simulink model "MPTC_TR"  (R2019b)
settings: Solver=ode4  StartTime=0.0  StopTime=1  FixedStep=1e-6  RelTol=1e-3  EnableMultiTasking=on
values from neighbouring files (symbols this model uses):
  B = 0    [Parameters_MPC.m]
  J = 0.0165    [Parameters_MPC.m]
  kr = (Lm/Lr)    (= 0.960714285714)    [Parameters_MPC.m]
  Lm = 0.0538    [Parameters_MPC.m]
  P = 2    [Parameters_MPC.m]
  r_sigma = Rs+Rr*(kr^2)    (= 0.445903864796)    [Parameters_MPC.m]
  Rs = 0.277    [Parameters_MPC.m]
  set_speed = 500    [Parameters_MPC.m]
  t_sigma = (sigma*Ls)/(r_sigma)    (= 0.00810392489023)    [Parameters_MPC.m]
  tr = Lr/Rr    (= 0.306010928962)    [Parameters_MPC.m]
libraries: powerlib_meascontrol x6, simulink x2, powerlib x1
settings Model: Creator=91913  LastModifiedBy=akhil
settings SolverCC: PositivePriorityOrder=on  AutoInsertRateTranBlk=on
settings DataIOCC: SaveOutput=off  DSMLogging=off  ReturnWorkspaceOutputs=off  SignalLoggingName=logsout_MPTCTR

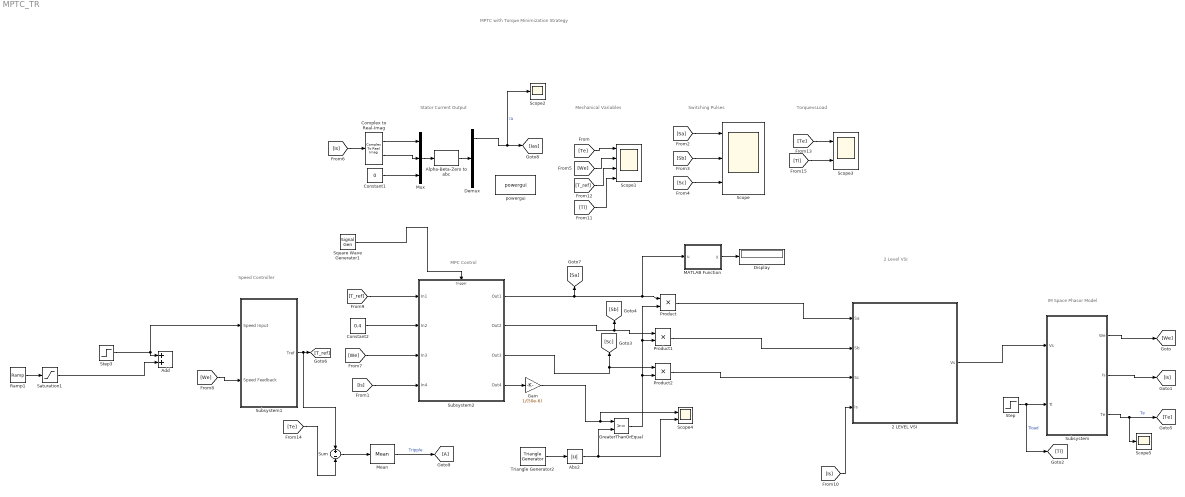
== system MPTC_TR ==
  note: MPTC with Torque Minimization Strategy
  note: IM Space Phasor Model
  note: 2 Level VSI
  note: Mechanical Variables
  note: Switching Pulses
  note: Speed Controller
  note: MPC Control
  note: Stator Current Output
  note: TorquevsLoad
  2 LEVEL VSI : Subsystem
  Abs2 : Abs
  Add : Sum
  Alpha-Beta-Zero to abc : powerlib_meascontrol/Transformations/Alpha-Beta-Zero to abc
      settings: SourceProductName=Simscape Electrical  SourceProductBaseCode=PS
  Complex to Real-Imag : ComplexToRealImag
  Constant1 : Constant  Value=0
  Constant2 : Constant  Value=0.4
  Demux : Demux  Outputs=3
  Display : Display
  Gain : Gain  Gain=1/(50e-6)
  GreaterThanOrEqual : RelationalOperator  OutDataTypeStr=boolean  RndMeth=Simplest
  MATLAB Function : MATLAB Function  TreatAsAtomicUnit=on
  Mean : powerlib_meascontrol/Measurements/Mean  Freq=41  Vinit=0  Ts=0
      settings: SourceProductName=Simscape Electrical
  Mux : Mux  Inputs=3
  Product : Product
  Product1 : Product
  Product2 : Product
  Ramp1 : simulink/Sources/Ramp  slope=-2*set_speed  start=0.4  InitialOutput=0
  Saturation1 : Saturate  UpperLimit=0  LowerLimit=-200
  Scope : Scope  NumInputPorts=3
  Scope1 : Scope  NumInputPorts=4
  Scope2 : Scope
  Scope3 : Scope  NumInputPorts=2
  Scope4 : Scope  NumInputPorts=2
  Scope5 : Scope
  Square Wave Generator1 : SignalGenerator  WaveForm=square  Frequency=1/(50e-6)
  Step : Step  Time=0.5  After=20  SampleTime=0
  Step3 : Step  Time=0.1  After=set_speed  SampleTime=0
  Subsystem : Subsystem
  Subsystem1 : Subsystem
  Subsystem2 : Subsystem
  Sum : Sum  Inputs=+-
  Triangle Generator2 : powerlib_meascontrol/Pulse & Signal Generators/Triangle Generator  Freq=5e4  Phase=90  Ts=0
      settings: SourceProductName=Simscape Electrical
  powergui : powerlib/powergui  Priority=1  SimulationMode=Continuous  SampleTime=50e-6  frequency=60  Iterations=50  frequencyindice=60  Pbase=100e6  ErrMax=1e-4  UnitsV=kV  UnitsW=MW  buscounter=0  FunctionMessages=off  echomessages=off  EnableUseOfTLC=off  CurrentSourceSwitches=off  DisableSnubberDevices=off  DisableRonSwitches=off  DisableVfSwitches=off  DisplayEquations=off  AutomaticDiscreteSolvers=off  SolverType=Tustin/Backward Euler (TBE)  Interpol=off  ExternalGateDelay=off  methode=off  Ts=100  x0status=blocks  SPID=on  SwTol=0  HookPort=off  NonlinearTolerance=1e-4  nMaxIteration=100  ContinueOnMaxIteration=off  RestoreLinks=warning  ResistiveCurrentMeasurement=off  Frange=[0:2:500]  Ylog=off  Xlog=on  ShowGrid=off  save=off  variable=ZData  structure=logsout  ZoomFFT=off  StartTime=1.2  cycles=20  DisplayStyle=1  fundamental=49.3  FreqAxis=on  MaxFrequency=1000  frequencyindicesteady=1  RmsSteady=1  display=off
      settings: SourceProductName=Simscape Electrical
  wires:
  2 LEVEL VSI/1(Vs) -> Subsystem/1(Vs)
  Gain/1 -> Scope4/1, GreaterThanOrEqual/1
  Square Wave Generator1/1 -> Subsystem2/Trigger
  [Tl] -> Scope3/2
  Subsystem/3(Te) -> Scope5/1, [Te]  "Te"
  Step/1 -> [Tl], Subsystem/2(Tl)  "Tload"
  Product/1 -> 2 LEVEL VSI/1(Sa)
  Triangle Generator2/1 -> Abs2/1
  Product1/1 -> 2 LEVEL VSI/2(Sb)
  Subsystem/1(We) -> [We]
  Subsystem2/4(Out4) -> Gain/1
  [Te] -> Scope3/1
  [Sc] -> Scope/3
  Subsystem2/2(Out2) -> Product1/1, [Sb]
  Product2/1 -> 2 LEVEL VSI/3(Sc)
  GreaterThanOrEqual/1 -> Product/2, Product1/2, Product2/2
  Constant1/1 -> Mux/3
  [Te] -> Scope1/1
  Subsystem2/3(Out3) -> [Sc], Product2/1
  Subsystem2/1(Out1) -> MATLAB Function/1(u), Product/1, [Sa]
  [Is] -> Subsystem2/4(In4)
  Complex to Real-Imag/2 -> Mux/2
  [Is] -> Complex to Real-Imag/1
  [Sa] -> Scope/1
  [We] -> Subsystem2/3(In3)
  Complex to Real-Imag/1 -> Mux/1
  Subsystem/2(Is) -> [Is]
  Abs2/1 -> Scope4/2, GreaterThanOrEqual/2
  [We] -> Scope1/2
  Alpha-Beta-Zero to abc/1 -> Demux/1
  [Tl] -> Scope1/4
  Subsystem1/1(Tref) -> Sum/1, [T_ref]
  Mux/1 -> Alpha-Beta-Zero to abc/1
  [We] -> Subsystem1/2(Speed Feedback)
  [T_ref] -> Scope1/3
  [Sb] -> Scope/2
  [Is] -> 2 LEVEL VSI/4(Is)
  Constant2/1 -> Subsystem2/2(In2)
  Demux/1 -> Scope2/1, [Ias]  "Ia"
  [Te] -> Sum/2
  Sum/1 -> Mean/1
  Mean/1 -> [A]  "Tripple"
  [T_ref] -> Subsystem2/1(In1)
  MATLAB Function/1(y) -> Display/1
  Step3/1 -> Subsystem1/1(Speed Input), Add/1
  Saturation1/1 -> Add/2
  Ramp1/1 -> Saturation1/1

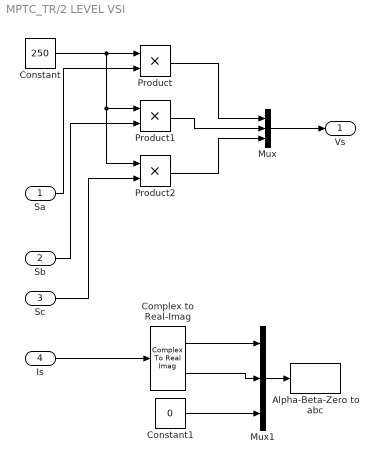
== system MPTC_TR/2 LEVEL VSI ==
  Sa : Inport
  Sb : Inport  Port=2
  Sc : Inport  Port=3
  Is : Inport  Port=4
  Alpha-Beta-Zero to abc : powerlib_meascontrol/Transformations/Alpha-Beta-Zero to abc
      settings: SourceProductName=Simscape Electrical  SourceProductBaseCode=PS
  Complex to Real-Imag : ComplexToRealImag
  Constant : Constant  Value=250
  Constant1 : Constant  Value=0
  Mux : Mux  Inputs=3
  Mux1 : Mux  Inputs=3
  Product : Product
  Product1 : Product
  Product2 : Product
  Vs : Outport
  wires:
  Sa/1 -> Product/2
  Sb/1 -> Product1/2
  Sc/1 -> Product2/2
  Constant/1 -> Product2/1, Product1/1, Product/1
  Product/1 -> Mux/1
  Product1/1 -> Mux/2
  Product2/1 -> Mux/3
  Mux/1 -> Vs/1
  Complex to Real-Imag/1 -> Mux1/1
  Complex to Real-Imag/2 -> Mux1/2
  Constant1/1 -> Mux1/3
  Mux1/1 -> Alpha-Beta-Zero to abc/1
  Is/1 -> Complex to Real-Imag/1

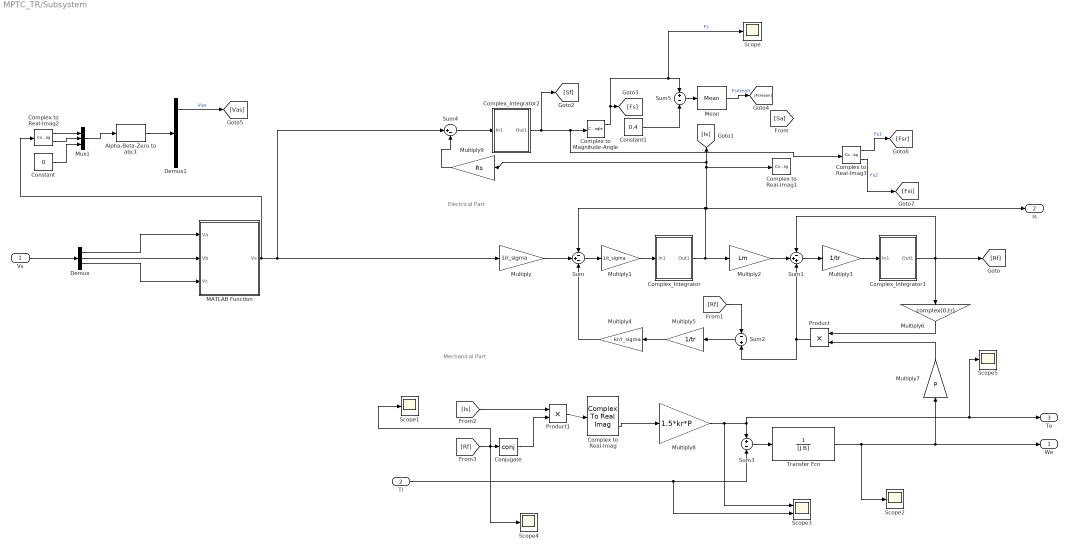
== system MPTC_TR/Subsystem ==
  note: Mechanical Part
  note: Electrical Part
  Vs : Inport
  Tl : Inport  Port=2
  Alpha-Beta-Zero to abc1 : powerlib_meascontrol/Transformations/Alpha-Beta-Zero to abc
      settings: SourceProductName=Simscape Electrical  SourceProductBaseCode=PS
  Complex to Magnitude-Angle : ComplexToMagnitudeAngle
  Complex to Real-Imag{,1..3} (4 alike) : ComplexToRealImag
  Complex_Integrator : Subsystem
  Complex_Integrator1 : Subsystem
  Complex_Integrator2 : Subsystem
  Conjugate : Math  Operator=conj  RndMeth=Zero  SaturateOnIntegerOverflow=on
  Constant : Constant  Value=0
  Constant1 : Constant  Value=0.4
  Demux : Demux  Outputs=3
  Demux1 : Demux  Outputs=3
  MATLAB Function : MATLAB Function  TreatAsAtomicUnit=on
  Mean : powerlib_meascontrol/Measurements/Mean  Freq=41  Vinit=0  Ts=0
      settings: SourceProductName=Simscape Electrical
  Multiply : Gain  Gain=1/r_sigma
  Multiply1 : Gain  Gain=1/t_sigma
  Multiply2 : Gain  Gain=Lm
  Multiply3 : Gain  Gain=1/tr
  Multiply4 : Gain  Gain=kr/r_sigma
  Multiply5 : Gain  Gain=1/tr
  Multiply6 : Gain  Gain=complex(0,tr)
  Multiply7 : Gain  Gain=P
  Multiply8 : Gain  Gain=1.5*kr*P
  Multiply9 : Gain  Gain=Rs
  Mux1 : Mux  Inputs=3
  Product : Product
  Product1 : Product
  Scope{,1..2,4..5} (5 alike) : Scope
  Scope3 : Scope  NumInputPorts=2
  Sum : Sum  Inputs=-+-
  Sum1 : Sum  Inputs=-++
  Sum2 : Sum  Inputs=-+
  Sum3 : Sum  Inputs=+-
  Sum4 : Sum  Inputs=|+-
  Sum5 : Sum  Inputs=+-
  Transfer Fcn : TransferFcn  Denominator=[J B]
  We : Outport
  Is : Outport  Port=2
  Te : Outport  Port=3
  wires:
  [Is] -> Product1/1
  Multiply1/1 -> Complex_Integrator/1(In1)
  Multiply4/1 -> Sum/3
  Multiply3/1 -> Complex_Integrator1/1(In1)
  Sum1/1 -> Multiply3/1
  Complex to Real-Imag/2 -> Multiply8/1
  Complex_Integrator1/1(Out1) -> Sum1/1, [Rf], Multiply6/1
  Tl/1 -> Scope3/2, Sum3/2
  Conjugate/1 -> Product1/2
  Multiply7/1 -> Product/2
  Multiply8/1 -> Scope3/1, Sum3/1, Scope5/1, Te/1
  Multiply2/1 -> Sum1/2
  Multiply/1 -> Sum/2
  Multiply6/1 -> Product/1
  Product/1 -> Sum2/2, Sum1/3
  Multiply5/1 -> Multiply4/1
  Sum2/1 -> Multiply5/1
  Transfer Fcn/1 -> Scope2/1, We/1, Multiply7/1
  Sum/1 -> Multiply1/1
  [Rf] -> Scope1/1, Conjugate/1, Scope4/1
  Product1/1 -> Complex to Real-Imag/1
  Sum3/1 -> Transfer Fcn/1
  [Rf] -> Sum2/1
  Sum4/1 -> Complex_Integrator2/1(In1)
  Complex_Integrator2/1(Out1) -> Complex to Real-Imag3/1, Complex to Magnitude-Angle/1, [Sf]
  Multiply9/1 -> Sum4/2
  Complex_Integrator/1(Out1) -> Multiply2/1, Multiply9/1, [Is], Complex to Real-Imag1/1, Is/1, Sum/1
  MATLAB Function/1(Vs) -> Complex to Real-Imag2/1, Sum4/1, Multiply/1
  Vs/1 -> Demux/1
  Demux/1 -> MATLAB Function/1(Va)
  Demux/2 -> MATLAB Function/2(Vb)
  Demux/3 -> MATLAB Function/3(Vc)
  Constant/1 -> Mux1/3
  Alpha-Beta-Zero to abc1/1 -> Demux1/1
  Mux1/1 -> Alpha-Beta-Zero to abc1/1
  Complex to Real-Imag2/2 -> Mux1/2
  Complex to Real-Imag2/1 -> Mux1/1
  Complex to Magnitude-Angle/1 -> Scope/1, Sum5/1, [Fs]  "Fs"
  Constant1/1 -> Sum5/2
  Sum5/1 -> Mean/1
  Mean/1 -> [Fsmean]  "Fsmean"
  Demux1/1 -> [Vas]  "Vas"
  Complex to Real-Imag3/2 -> [Fsi]  "Fs2"
  Complex to Real-Imag3/1 -> [Fsr]  "Fs1"

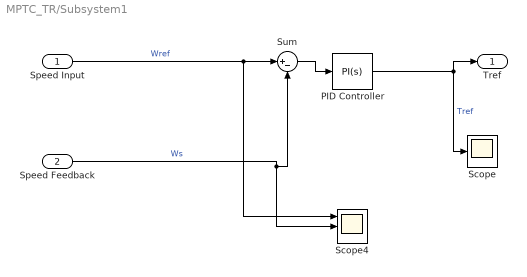
== system MPTC_TR/Subsystem1 ==
  Speed Input : Inport
  Speed Feedback : Inport  Port=2
  PID Controller : simulink/Continuous/PID Controller  Controller=PI  Form=Parallel  TimeDomain=Continuous-time  SampleTime=-1  IntegratorMethod=Forward Euler  FilterMethod=Forward Euler  ControllerParametersSource=internal  P=100  I=2000  D=0  UseFilter=on  N=100  TunerSelectOption=Transfer Function Based (PID Tuner App)  InitialConditionSource=internal  InitialConditionForIntegrator=0  InitialConditionForFilter=0  DifferentiatorICPrevScaledInput=0  ExternalReset=none  TrackingMode=off  Kt=1  LimitOutput=on  UpperSaturationLimit=75  LowerSaturationLimit=-75  LinearizeAsGain=off  AntiWindupMode=clamping  Kb=1  POutMin=[]  POutMax=[]  IOutMin=[]  IOutMax=[]  DOutMin=[]  DOutMax=[]  NOutMin=[]  NOutMax=[]  SumOutMin=[]  SumOutMax=[]  SaturationOutMin=[]  SaturationOutMax=[]  PParamMin=[]  PParamMax=[]  IParamMin=[]  IParamMax=[]  DParamMin=[]  DParamMax=[]  NParamMin=[]  NParamMax=[]  KbParamMin=[]  KbParamMax=[]  KtParamMin=[]  KtParamMax=[]  KbOutMin=[]  KbOutMax=[]  KtOutMin=[]  KtOutMax=[]  IntegratorOutMin=[]  IntegratorOutMax=[]  FilterOutMin=[]  FilterOutMax=[]  SumI1OutMin=[]  SumI1OutMax=[]  SumI2OutMin=[]  SumI2OutMax=[]  SumI3OutMin=[]  SumI3OutMax=[]  SumI4OutMin=[]  SumI4OutMax=[]  SumDOutMin=[]  SumDOutMax=[]  DifferentiatorOutMin=[]  DifferentiatorOutMax=[]  FilterDiffOutCoefMin=[]  FilterDiffOutCoefMax=[]  ReciprocalOutMin=[]  ReciprocalOutMax=[]  SumDenOutMin=[]  SumDenOutMax=[]  SumNumOutMin=[]  SumNumOutMax=[]  DivideOutMin=[]  DivideOutMax=[]  IntegratorContinuousStateAttributes=''  IntegratorStateMustResolveToSignalObject=off  IntegratorRTWStateStorageClass=Auto  FilterContinuousStateAttributes=''  FilterStateMustResolveToSignalObject=off  FilterRTWStateStorageClass=Auto  ParallelPVariant=InternalParameters  IdealPVariant=Disabled  IVariant=InternalParameters  DVariant=Disabled  IntegratorVariant=Continuous  SatVariant=Enabled  AWVariant=ContClampingParallel  PCopyVariant=Disabled  TRVariant=Disabled  FdbkBlocksVariant=Forward  IdealPFdbkVariant=Disabled  SatFdbkVariant=Disabled  DerivativeFilterVariant=Disabled  NVariant=Disabled  NCopyVariant=Disabled_SignalSpec  FilterICVariant=Disabled  IntegratorICVariant=InternalICs  ExternalResetVariant=Disabled  TRSumVariant=Passthrough  SumFdbkVariant=Disabled  SumVariant=Sum_PI
  Scope : Scope
  Scope4 : Scope  NumInputPorts=3
  Sum : Sum  Inputs=|+-
  Tref : Outport
  wires:
  Speed Input/1 -> Scope4/1, Sum/1  "Wref"
  Speed Feedback/1 -> Scope4/2, Sum/2  "Ws"
  Sum/1 -> PID Controller/1
  PID Controller/1 -> Tref/1, Scope/1  "Tref"

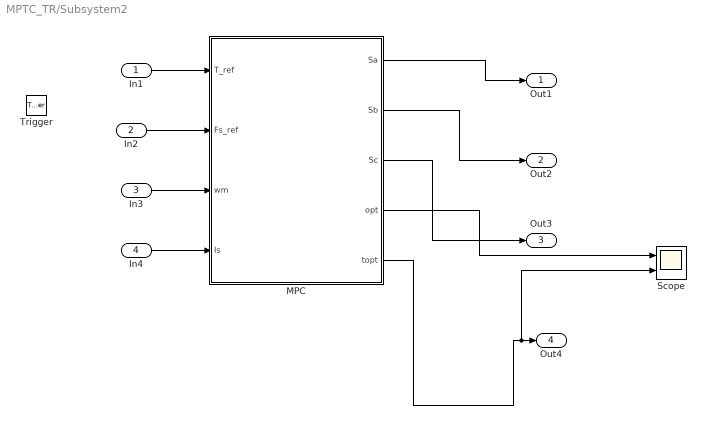
== system MPTC_TR/Subsystem2 ==
  In1 : Inport
  In2 : Inport  Port=2
  In3 : Inport  Port=3
  In4 : Inport  Port=4
  Trigger : TriggerPort  VariantControl=Variant  ShowOutputPort=on  PortDimensions=1
  MPC : MATLAB Function  TreatAsAtomicUnit=on
  Scope : Scope  NumInputPorts=2
  Out1 : Outport
  Out2 : Outport  Port=2
  Out3 : Outport  Port=3
  Out4 : Outport  Port=4
  wires:
  In4/1 -> MPC/4(Is)
  In3/1 -> MPC/3(wm)
  MPC/2(Sb) -> Out2/1
  MPC/1(Sa) -> Out1/1
  MPC/3(Sc) -> Out3/1
  In1/1 -> MPC/1(T_ref)
  In2/1 -> MPC/2(Fs_ref)
  MPC/5(topt) -> Scope/2, Out4/1
  MPC/4(opt) -> Scope/1

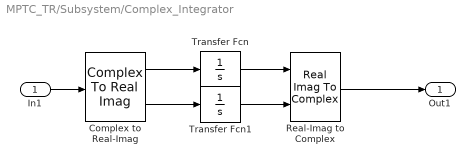
== system MPTC_TR/Subsystem/Complex_Integrator ==
  In1 : Inport
  Complex to Real-Imag : ComplexToRealImag
  Real-Imag to Complex : RealImagToComplex
  Transfer Fcn : TransferFcn  Denominator=[1 0]
  Transfer Fcn1 : TransferFcn  Denominator=[1 0]
  Out1 : Outport
  wires:
  In1/1 -> Complex to Real-Imag/1
  Complex to Real-Imag/1 -> Transfer Fcn/1
  Complex to Real-Imag/2 -> Transfer Fcn1/1
  Transfer Fcn/1 -> Real-Imag to Complex/1
  Transfer Fcn1/1 -> Real-Imag to Complex/2
  Real-Imag to Complex/1 -> Out1/1

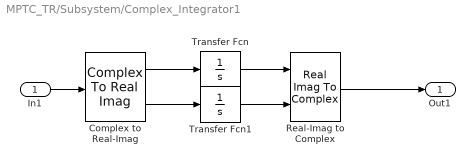
== system MPTC_TR/Subsystem/Complex_Integrator1 ==
  In1 : Inport
  Complex to Real-Imag : ComplexToRealImag
  Real-Imag to Complex : RealImagToComplex
  Transfer Fcn : TransferFcn  Denominator=[1 0]
  Transfer Fcn1 : TransferFcn  Denominator=[1 0]
  Out1 : Outport
  wires:
  In1/1 -> Complex to Real-Imag/1
  Complex to Real-Imag/1 -> Transfer Fcn/1
  Complex to Real-Imag/2 -> Transfer Fcn1/1
  Transfer Fcn/1 -> Real-Imag to Complex/1
  Transfer Fcn1/1 -> Real-Imag to Complex/2
  Real-Imag to Complex/1 -> Out1/1

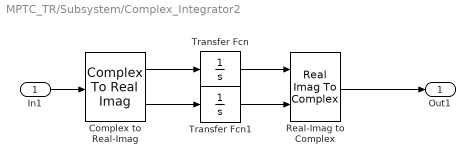
== system MPTC_TR/Subsystem/Complex_Integrator2 ==
  In1 : Inport
  Complex to Real-Imag : ComplexToRealImag
  Real-Imag to Complex : RealImagToComplex
  Transfer Fcn : TransferFcn  Denominator=[1 0]
  Transfer Fcn1 : TransferFcn  Denominator=[1 0]
  Out1 : Outport
  wires:
  In1/1 -> Complex to Real-Imag/1
  Complex to Real-Imag/1 -> Transfer Fcn/1
  Complex to Real-Imag/2 -> Transfer Fcn1/1
  Transfer Fcn/1 -> Real-Imag to Complex/1
  Transfer Fcn1/1 -> Real-Imag to Complex/2
  Real-Imag to Complex/1 -> Out1/1

== matlab function MPTC_TR/Subsystem2/MPC ==
  settings: updateMethod=DISCRETE
  data: T_ref input; Sa output; Fs_ref input; wm input; Is input; Sb output; Sc output; opt output; topt output
function [Sa,Sb,Sc,opt,topt]   = MPC(T_ref,Fs_ref,wm,Is)

Ts=50e-6;%Sampling time or Time Window for Kth sample
%Supply DC Voltage
Vdc=250;
%Machine Parameters
Rs=0.277;
Rr=0.183;
Lr=0.056;
Ls=0.0553;
Lm=0.0538;
P=2;%pole pairs
Fs_nom=0.4;
T_nom=25;
Is_nom=25;
%Electrical Time Constants
tr=Lr/Rr;
%Constants in equation
sigma=(1-(Lm^2)/(Ls*Lr));
kr=(Lm/Lr);
r_sigma=Rs+Rr*(kr^2);
t_sigma=(sigma*Ls)/(r_sigma);
lambda=1/((Ls*Lr)-Lm^2);
%weight=T_nom/Fs_nom;
%Voltage vectors
V0=0;
V1=complex((2/3)*Vdc,0);
V2=complex((1/3)*Vdc,(sqrt(3)/3)*Vdc);
V3=complex((-1/3)*Vdc,(sqrt(3)/3)*Vdc);
V4=-V1;
V5=-V2;
V6=-V3;
V7= V0;
V=[V0 V1 V2 V3 V4 V5 V6 V7];
%Switching States

states=[0 0 0;1 0 0;1 1 0;0 1 0;0 1 1;0 0 1;1 0 1;1 1 1];

persistent x_opt Fs%since previous values are required for prediction and estimation
if isempty(x_opt)
    x_opt=2;
end
if isempty(Fs)
    Fs=complex(0,0);
end

%stator flux estimate
Fs=Fs+Ts*(V(x_opt)-(Rs*Is));
%Rotor Flux estimate
Fr=((Lr/Lm)*Fs)+(Is*(Lm-(Lr*Ls/Lm)));
% [theta, rho] = cart2pol(real(Fr), imag(Fr));
cost_opt=1e14;
topt=Ts;

%Prediction of stator current,flux vectors and Torque for each voltage
%vectors
V_opt=complex(1,0);
A=(Rs/(sigma*Ls))+(Rr/(sigma*Lr));
B=(1.5*P)*(Lm/(sigma*Ls*Lr));
Te=(3/2)*P*imag(conj(Fs)*Is);
S0=(-Te*A)-(B*imag(complex(0,wm*P)*Fs*conj(Fr)));
for loop=1:8
    V_loop=V(loop);% iterative voltage vector
     %Stator current prediction
    Isp=Is*(t_sigma/(Ts+t_sigma))+(Ts/(t_sigma+Ts))*(1/r_sigma)*(Fr*((kr/tr)-complex(0,P*wm*kr))+V_loop);
    %Stator flux prediction based on discretization
    Fsp=Fs+(Ts*V_loop)-Rs*Ts*Isp;
   
    %Torque prediction
    Tp=(3/2)*P*imag(conj(Fsp)*Isp);

     f=0;
     if abs(Isp) > Is_nom  
           f = 1e14; 
     end
     %cost=34*(abs(Fs_ref-abs(Fsp))/Fs_nom);  
     %cost=(abs(T_ref-Tp))+100*(abs(Fs_ref-abs(Fsp)));
     cost=1.25*(abs(T_ref-Tp)/T_nom)+5*(abs(Fs_ref-abs(Fsp))/Fs_nom)+f;
      %cost=abs(Fsref-Fsp);
     if(cost<cost_opt) 
     x_opt=loop;
     cost_opt=cost;
     V_opt=V_loop;
     end     
end
S1=S0+(B*imag(V_opt*conj(Fr)));
%Outpt switching states
Sa=states(x_opt,1);
Sb=states(x_opt,2);
Sc=states(x_opt,3); 
t_opt=((2*(T_ref-Te))-(S0*Ts))/(2*S1-S0);
topt=t_opt;

if(t_opt<0&& abs(t_opt)>Ts)
    topt=Ts;
end
if(t_opt<0&& abs(t_opt)<Ts)
   topt=0;
end    
  
if (t_opt>Ts)
    topt=Ts;
end    
topt=Ts;
opt=x_opt;

== matlab function MPTC_TR/Subsystem/MATLAB Function ==
  data: Va input; Vs output; Vb input; Vc input
function Vs = fcn(Va,Vb,Vc)

a=complex(cos(2*pi/3),sin(2*pi/3)); 
Vs =(2/3)*(Va+(a*Vb)+((a^2)*Vc)) ;

== matlab function MPTC_TR/MATLAB Function ==
  data: u input; y output
function y = fcn(u)
persistent count prestate;
if(isempty(count))
    count=0;
end    
if(isempty(prestate))
    prestate=0;
end  
if(u~=prestate)
count=count+1;    
end
prestate=u;
y=count;
